simulink model "Jaccobi"  (R2020a)
settings: Solver=VariableStepAuto  StartTime=0.0  StopTime=10.0  RelTol=1e-3
libraries: simulink x5, roblocks x2
settings Model: Creator=hemingshan  LastModifiedBy=hemingshan

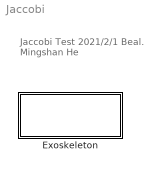
== system Jaccobi ==
  note: Jaccobi Test
      | 2021/2/1
      | Beal. Mingshan He
  Exoskeleton : Subsystem
      mask Display: disp('Jaccobi')

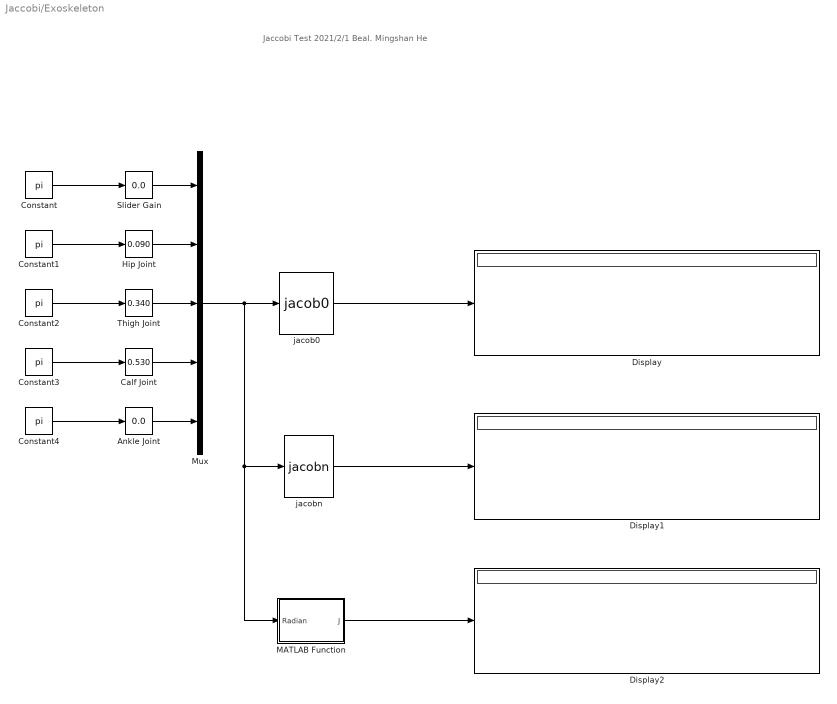
== system Jaccobi/Exoskeleton ==
  note: Jaccobi Test
      | 2021/2/1
      | Beal. Mingshan He
  Ankle Joint : simulink/Math Operations/Slider Gain  gain=0.0  low=0  high=0.5
  Calf Joint : simulink/Math Operations/Slider Gain  gain=0.530  low=0  high=1
  Constant{,1..4} (5 alike) : Constant  Value=pi
  Display : Display
  Display1 : Display
  Display2 : Display
  Hip Joint : simulink/Math Operations/Slider Gain  gain=0.090  low=0  high=0.5
  MATLAB Function : MATLAB Function  TreatAsAtomicUnit=on
  Mux : Mux  Inputs=5
  Slider Gain : simulink/Math Operations/Slider Gain  gain=0.0  low=0  high=2
  Thigh Joint : simulink/Math Operations/Slider Gain  gain=0.340  low=0  high=1
  "jacob0 " : roblocks/Arm/jacob0   robot=robot
  jacobn : roblocks/Arm/jacobn  robot=robot
  wires:
  Constant3/1 -> Calf Joint/1
  Constant2/1 -> Thigh Joint/1
  Hip Joint/1 -> Mux/2
  Thigh Joint/1 -> Mux/3
  Calf Joint/1 -> Mux/4
  Slider Gain/1 -> Mux/1
  Ankle Joint/1 -> Mux/5
  Constant1/1 -> Hip Joint/1
  Constant/1 -> Slider Gain/1
  Constant4/1 -> Ankle Joint/1
  Mux/1 -> MATLAB Function/1(Radian), jacobn/1, "jacob0 "/1
  "jacob0 "/1 -> Display/1
  jacobn/1 -> Display1/1
  MATLAB Function/1(J) -> Display2/1

== matlab function Jaccobi/Exoskeleton/MATLAB Function ==
  data: Radian input; J output
function J = Jaccobi(Radian)
%%计算基坐标下的雅可比矩阵
%% input 
theta1 = Radian(2);
theta2 = Radian(3);
theta3 = Radian(4);
theta4 = Radian(5);
%% D-H parameters 
d1 = -0.097;
a3 = -sqrt(0.23966^2+0.28189^2);
a4 = -sqrt(-0.15989^2+0.31135^2);
Tbase = [1,0,0,0;0,1,0,0;0,0,1,d1;0,0,0,1];
T1=[1,0,0,0;0,1,0,0;0,0,1,0;0,0,0,1];
T2=[cos(theta1),-sin(theta1),0,0;sin(theta1),cos(theta1),0,0;0,0,1,0;0,0,0,1];
T3=[cos(theta2),-sin(theta2),0,0;0,0,-1,0;sin(theta2),cos(theta2),0,0;0,0,0,1];
T4=[cos(theta3),-sin(theta3),0,a3;sin(theta3),cos(theta3),0,0;0,0,1,0;0,0,0,1];
Ttool = [cos(theta4),-sin(theta4),0,a4;sin(theta4),cos(theta4),0,0;0,0,1,0;0,0,0,1];
%% Tbase T1~T6 Ttool
% KPS44=Tbase*T1*T2*T3*T4*T5*T6*Ttool;
%k7=Ttool;
k = zeros(4,4,4);
k(:,:,4)=Ttool;
k(:,:,3)=T4*Ttool;
k(:,:,2)=T3*T4*Ttool;
k(:,:,1)=T2*T3*T4*Ttool;
Jn=zeros(6,4);
for i=1:4
    Jn(1,i)=-k(1,1,i)*k(2,4,i)+k(2,1,i)*k(1,4,i);
    Jn(2,i)=-k(1,2,i)*k(2,4,i)+k(2,2,i)*k(1,4,i);
    Jn(3,i)=-k(1,3,i)*k(2,4,i)+k(2,3,i)*k(1,4,i);
    Jn(4,i)=k(3,1,i);
    Jn(5,i)=k(3,2,i);
    Jn(6,i)=k(3,3,i);
end
FK = Tbase * T1 * T2 * T3 * T4 * Ttool;
FK66 = FK(1:3,1:3);
RR = [ FK66 zeros(3,3);
       zeros(3,3) FK66];
Jn_Base = RR*Jn;
J = Jn;
